simulink model "xpcasyncbuffer"  (Simulink 6.0)
settings: Solver=FixedStepDiscrete  StartTime=0.0  StopTime=inf  FixedStep=0.001  RelTol=1e-3
libraries: xpclib x4
settings Model: Creator=mvetsch  LastModifiedBy=ekbas  ExtModeTrigMode=oneshot  ExtModeArmWhenConnect=off  BufferReuse=off
settings DataIOCC: LimitDataPoints=off  SaveState=on  SignalLoggingName=logsOut
settings OptimizationCC: BlockReduction=off  BooleanDataType=off  InlineInvariantSignals=off  OptimizeBlockIOStorage=off  BufferReuse=off  EnforceIntegerDowncast=off  FoldNonRolledExpr=off  LocalBlockOutputs=off
settings DebuggingCC: CheckExecutionContextPreStartOutputMsg=on  CheckExecutionContextRuntimeOutputMsg=on  SolverPrmCheckMsg=none  MultiTaskRateTransMsg=warning
settings RTWCC: SystemTargetFile=xpctarget.tlc  TemplateMakefile=xpc_default_tmf  Description=xPC Target  ProcessScript=xpctarget_make_rtw_hook
settings xpcTargetCC: TargetFcnLib=ansi_tfl_tmw.mat  GenFloatMathFcnCalls=ANSI_C  ModelReferenceCompliant=off  LifeSpan=inf
settings SFSimCC: SFSimApplyToAllLibs=on  SFSimBuildMode=Incremental

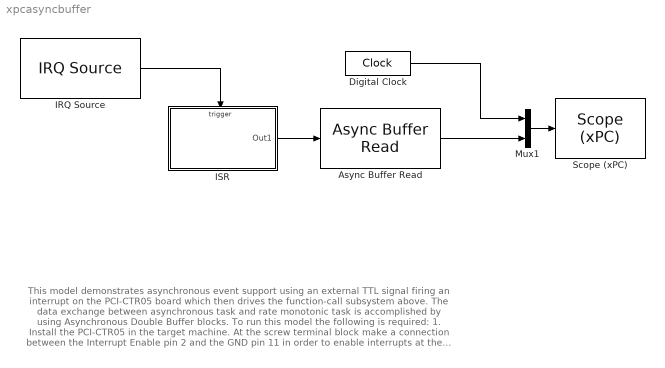
== system xpcasyncbuffer ==
  note: This model demonstrates asynchronous event support using an external TTL signal firing
      | an interrupt on the PCI-CTR05 board which then drives the function-call subsystem above.
      | The data exchange between asynchronous task and rate monotonic task is accomplished
      |  by using Asynchronous Double Buffer blocks.
      |
      | To run this model the following is required:
      |
      | 1. Install the PCI-CTR05 in the target machine. At the screw terminal block make a connection
      | between the Interrupt Enable pin 2 and the GND pin 11 in order to enable interrupts at the
      | board level. Then connect Interrupt Input pin 1 and GND pin 11 to a external TTL signal
      | source like a Pulse Generator. During execution of the target application the function-call
      | subsystem will then be executed whenever a TTL low-high signal transition occurs.
      |
      | 2. If not yet done, boot the target as an xPC Target machine. At the MATLAB command
      | prompt initiate command "getxpcpci" to list all PCI-boards present in the system.
      | Look up the IRQ line assigned to the PCI-CTR05 board and select this same IRQ
      | line in the IRQ Source block above. Then build the target application.
  Async Buffer Read : xpclib/Asynchronous Event/Async Buffer Read  sample_time=0.001
  Digital Clock : DigitalClock  SampleTime=0.001
  IRQ Source : xpclib/Asynchronous Event/IRQ Source  irqNo=5  preempt=on  b_type=CB PCI-CTR05  slot=-1
  ISR : Subsystem  TreatAsAtomicUnit=on  PropExecContextAcrossSSBoundary=on
  Mux1 : Mux  Inputs=2
  "Scope (xPC) " : xpclib/Misc./Scope (xPC)   scopeno=1  scopetype=Target  autostart=on  viewmode=Numerical  formatstr='%15.6f'  grid=on  ylimits=[0,0]  nosamples=3  noprepostsamples=0  interleave=1  triggermode=FreeRun  triggersignal=1  triggerlevel=0.0  triggerslope=Either  triggerscope=1  triggersample=0  filename=data.dat  mode=Lazy  writesize=512  autorestart=off
  wires:
  IRQ Source/1 -> ISR/Trigger
  Digital Clock/1 -> Mux1/1
  Mux1/1 -> "Scope (xPC) "/1
  ISR/1(Out1) -> Async Buffer Read/1
  Async Buffer Read/1 -> Mux1/2

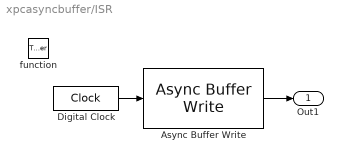
== system xpcasyncbuffer/ISR ==
  function : TriggerPort  TriggerType=function-call
  Async Buffer Write : xpclib/Asynchronous Event/Async Buffer Write  sample_time=-1
  Digital Clock : DigitalClock  SampleTime=-1
  Out1 : Outport
  wires:
  Digital Clock/1 -> Async Buffer Write/1
  Async Buffer Write/1 -> Out1/1
